simulink model "model0"  (R2018b)
settings: Solver=ode4  StartTime=0.0  StopTime=10.0  FixedStep=0.01  RelTol=1e-3
values from neighbouring files (symbols this model uses):
  K = 1/(R*C)    (= 1)    [script.m]
  WPC = 4    [script.m]
settings Model: Creator=student  LastModifiedBy=student

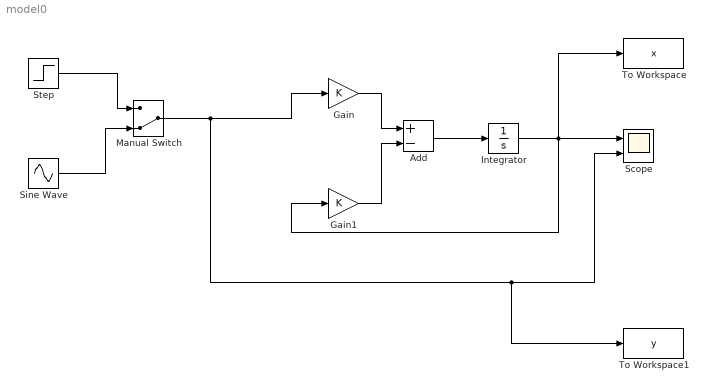
== system model0 ==
  Add : Sum  Inputs=+-
  Gain : Gain  Gain=K
  Gain1 : Gain  Gain=K
  Integrator : Integrator  InitialCondition=WPC
  Manual Switch : ManualSwitch  CurrentSetting=0
  Scope : Scope  NumInputPorts=2
  Sine Wave : Sin  Frequency=10*2*pi  SampleTime=0
  Step : Step  After=0  SampleTime=0
  To Workspace : ToWorkspace  VariableName=x  SampleTime=-1
  To Workspace1 : ToWorkspace  VariableName=y  SampleTime=-1
  wires:
  Step/1 -> Manual Switch/1
  Sine Wave/1 -> Manual Switch/2
  Manual Switch/1 -> To Workspace1/1, Scope/2, Gain/1
  Gain/1 -> Add/1
  Gain1/1 -> Add/2
  Add/1 -> Integrator/1
  Integrator/1 -> To Workspace/1, Gain1/1, Scope/1
